simulink library "drc"  (Simulink 8.1)
settings: Solver=ode1  StartTime=0.0  StopTime=Inf  FixedStep=0.001  RelTol=1e-3
PostLoadFcn:
  | , if any(exist('dsrtsu_mdlpostloadfcn', 'file') == [2, 3, 6]), try dsrtsu_mdlpostloadfcn('Execute', bdroot); catch fprintf('Error in PostLoadFcn (dsrtsu_mdlpostloadfcn) for model "%s":\n %s\n', bdroot, lasterr); end, end,
undefined symbols (not defined in the file or in its folder): AACC_VehSpdError_kph, MACC_ACCLookUpDecel_mps2, ZERO_FLOAT
libraries: hcu_lib x1
settings Model: DSRTSU_INTERNAL_RTI_VER=450  DSRTSU_INTERNAL_RTI_TYPE=rti1401  RTICANMMDATA=struct('GeneralSetupData',struct('modelroot','D:\ELN150201_TAIWAN\trunk\AdasDragon\software\sw_development\arch\app\acc','generalsettings',struct('filesettings',struct('destfolder',struct('Name','RTICANMM_FILES','Check',1),'buildfolder',struct('Name','.','Check',1),'AbsDestfolder',struct('Name','D:\ELN150201_TAIWAN\trunk\AdasDragon\software\sw_development\arch\app\acc\RTICANMM_FILES'),'AbsBuildfolder',struct('Name','D:\ELN150201_TAIWAN\trunk\AdasDragon\software\sw_development\arch\app\acc'))),'options',struct('addpaths',1,'rmpaths',1,'addtrcexclusion',logical(1),'cannavigator',struct('checkmonitoring',0),'show_usrtrc',0,'use_usrtrc',0),'advanced',struct('options',[1 1 1 1 1 1 1 1 1 1 1 1 1 1 1 1 1 1 1 1 1 1 1 1 1 1 1 1 1 1 1 1 1 1 1 1 1 1 1 1 1 1 1 1 1 1 1 1 1 1 1 1 1 1 1 1 1 1 1 1 1 1 1 1 1 1 1 1 1 1 1 1 1 1 1 1 1 1 1 1 1 1 1 1 1 1 1 1 1 1 1 1 1 1 1 1 1 1 1 1]),'MPSetup',{{}},'modelname','drd','block','drd'))  DSRTSU_INTERNAL_RTIFPGA=40  Creator=AT015555  LastModifiedBy=AT015555

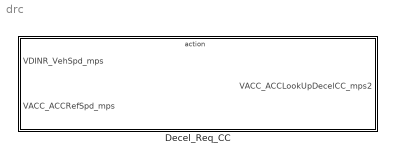
== system drc ==
  Decel_Req_CC : Subsystem  TreatAsAtomicUnit=on

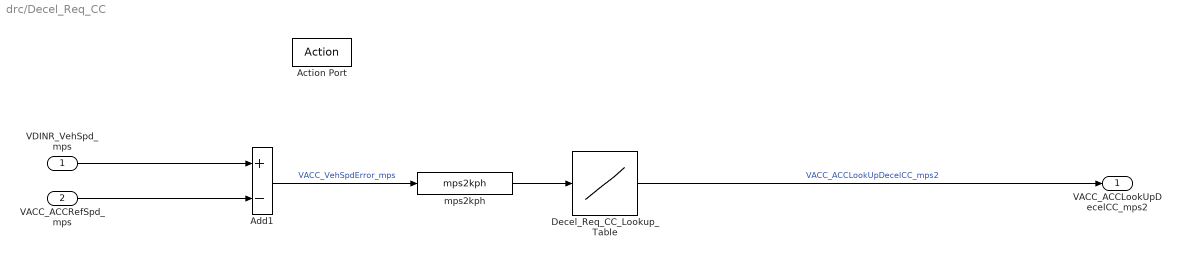
== system drc/Decel_Req_CC ==
  VDINR_VehSpd_mps : Inport
  VACC_ACCRefSpd_mps : Inport  Port=2
  Action Port : ActionPort
  Add1 : Sum  Inputs=+-
  Decel_Req_CC_Lookup_Table : Lookup_n-D  NumberOfTableDimensions=1  BreakpointsForDimension1=AACC_VehSpdError_kph  Table=MACC_ACCLookUpDecel_mps2  ExtrapMethod=Clip  UseLastTableValue=on  RndMeth=Simplest  InputSameDT=on
  mps2kph : hcu_lib/mps2kph
  VACC_ACCLookUpDecelCC_mps2 : Outport  OutputWhenDisabled=reset  InitialOutput=ZERO_FLOAT
  wires:
  VDINR_VehSpd_mps/1 -> Add1/1
  Add1/1 -> mps2kph/1  "VACC_VehSpdError_mps"
  VACC_ACCRefSpd_mps/1 -> Add1/2
  Decel_Req_CC_Lookup_Table/1 -> VACC_ACCLookUpDecelCC_mps2/1  "VACC_ACCLookUpDecelCC_mps2"
  mps2kph/1 -> Decel_Req_CC_Lookup_Table/1
